simulink model "task2_book"  (R2017a)
settings: Solver=VariableStepAuto  StartTime=0.0  StopTime=400  MaxStep=1e-4*w_base  RelTol=1e-3
settings Model: Creator=Oskar  LastModifiedBy=Callum

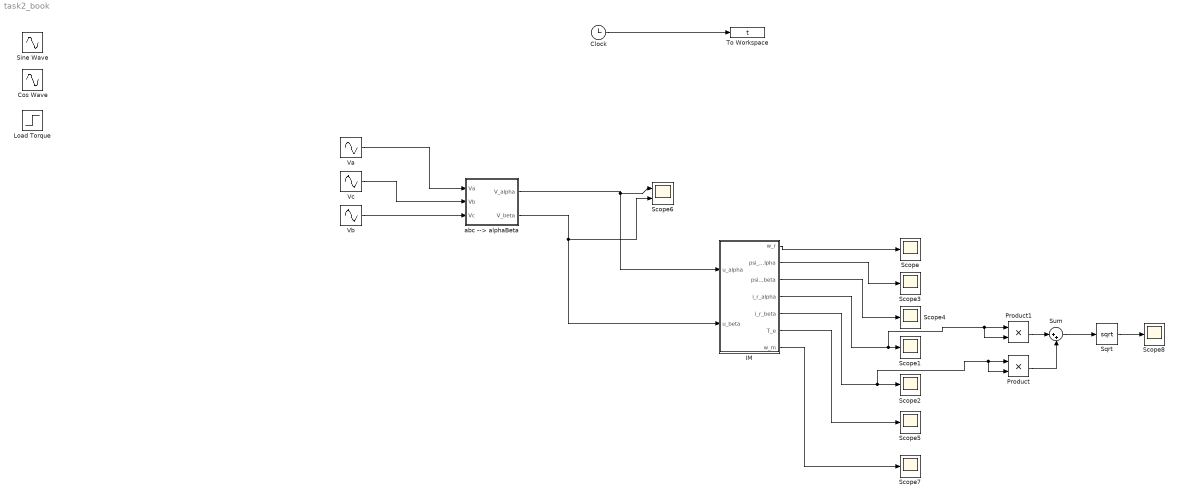
== system task2_book ==
  Clock : Clock
  Cos Wave : Sin  Phase=pi/2  SampleTime=0
  IM : Subsystem  mask{RR=0.02, RS=0.04, LM=2, Ls=0.2, J=100, p=1, b_w1=0.8, b_w2=0}
      mask prompts: RR "Rr [p.u]"; RS "Rs [p.u]"; LM "Lm [p.u]"; Ls "Ls [p.u]"; J "J [p.u]"
  Load Torque : Step  Time=0.3  After=0.3  SampleTime=0
  Product : Product
  Product1 : Product
  Scope{,1..5,7..8} (8 alike) : Scope
  Scope6 : Scope  NumInputPorts=2
  Sine Wave : Sin  SampleTime=0
  Sqrt : Sqrt  SaturateOnIntegerOverflow=on
  Sum : Sum  Inputs=|++
  To Workspace : ToWorkspace  VariableName=t
      settings: MaxDataPoints=10000000
  Va : Sin  Amplitude=sqrt(2)  SampleTime=0
  Vb : Sin  Amplitude=sqrt(2)  Phase=2*pi/3  SampleTime=0
  Vc : Sin  Amplitude=sqrt(2)  Phase=4*pi/3  SampleTime=0
  abc --> alphaBeta : Subsystem
  wires:
  IM/1(w_r) -> Scope/1
  IM/4(i_r_alpha) -> Product1/2, Product1/1, Scope1/1
  IM/5(i_r_beta) -> Product/2, Product/1, Scope2/1
  IM/2(psi_r_alpha) -> Scope3/1
  IM/3(psi_r_beta) -> Scope4/1
  IM/6(T_e) -> Scope5/1
  Va/1 -> abc --> alphaBeta/1(Va)
  abc --> alphaBeta/1(V_alpha) -> Scope6/1, IM/1(u_alpha)
  abc --> alphaBeta/2(V_beta) -> Scope6/2, IM/2(u_beta)
  Vc/1 -> abc --> alphaBeta/2(Vb)
  Vb/1 -> abc --> alphaBeta/3(Vc)
  Clock/1 -> To Workspace/1
  IM/7(w_m) -> Scope7/1
  Product/1 -> Sum/2
  Product1/1 -> Sum/1
  Sum/1 -> Sqrt/1
  Sqrt/1 -> Scope8/1

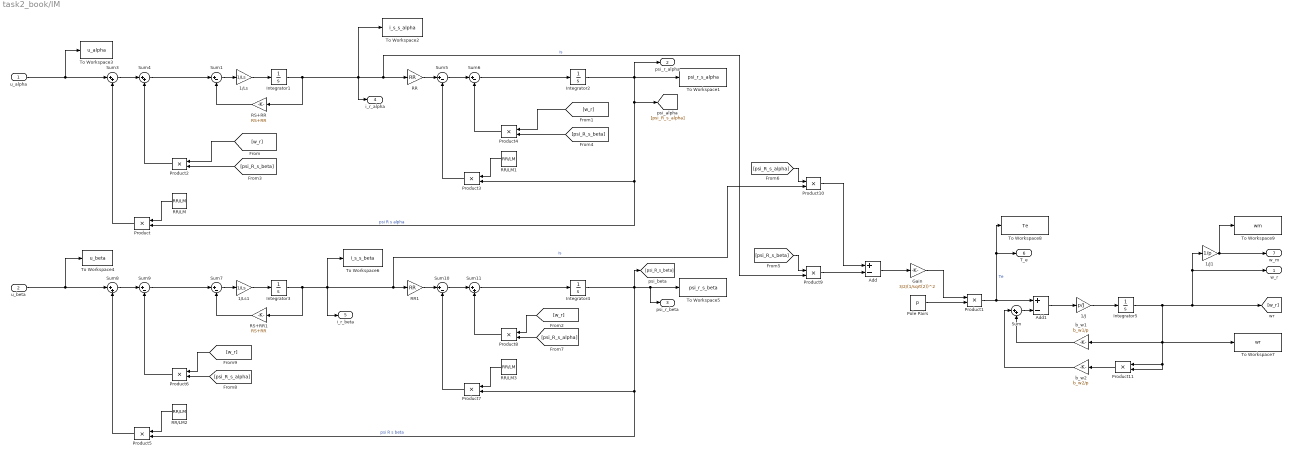
== system task2_book/IM ==
  u_alpha : Inport
  u_beta : Inport  Port=2
  1/J : Gain  Gain=p/J
  1/J1 : Gain  Gain=1/p
  1/Ls : Gain  Gain=1/Ls
  1/Ls1 : Gain  Gain=1/Ls
  Add : Sum  Inputs=+-
  Add1 : Sum  Inputs=+-
  Gain : Gain  Gain=3/2/(1/sqrt(2))^2
  Integrator{1..5} (5 alike) : Integrator
  Pole Pairs : Constant  Value=p
  Product{,1..11} (12 alike) : Product  SaturateOnIntegerOverflow=on  InputSameDT=on  OutDataTypeStr=Inherit: Same as first input
  RR : Gain  Gain=RR
  RR/LM{,1..3} (4 alike) : Constant  Value=RR/LM
  RR1 : Gain  Gain=RR
  RS+RR : Gain  Gain=RS+RR
  RS+RR1 : Gain  Gain=RS+RR
  Sum{,3..4,8,11} (5 alike) : Sum  Inputs=|++
  Sum{1,5..7,9..10} (6 alike) : Sum  Inputs=|+-
  To Workspace1 : ToWorkspace  VariableName=psi_r_s_alpha
      settings: MaxDataPoints=100000
  To Workspace2 : ToWorkspace  VariableName=i_s_s_alpha
      settings: MaxDataPoints=100000
  To Workspace3 : ToWorkspace  VariableName=u_alpha
      settings: MaxDataPoints=100000
  To Workspace4 : ToWorkspace  VariableName=u_beta
      settings: MaxDataPoints=100000
  To Workspace5 : ToWorkspace  VariableName=psi_r_s_beta
      settings: MaxDataPoints=100000
  To Workspace6 : ToWorkspace  VariableName=i_s_s_beta
      settings: MaxDataPoints=100000
  To Workspace7 : ToWorkspace  VariableName=wr
      settings: MaxDataPoints=100000
  To Workspace8 : ToWorkspace  VariableName=Te
      settings: MaxDataPoints=100000
  To Workspace9 : ToWorkspace  VariableName=wm
      settings: MaxDataPoints=100000
  b_w1 : Gain  Gain=b_w1/p
  b_w2 : Gain  Gain=b_w2/p
  w_r : Outport
  psi_r_alpha : Outport  Port=2
  psi_r_beta : Outport  Port=3
  i_r_alpha : Outport  Port=4
  i_r_beta : Outport  Port=5
  T_e : Outport  Port=6
  w_m : Outport  Port=7
  wires:
  RR/LM1/1 -> Product3/1
  Product3/1 -> Sum5/2
  [psi_R_s_alpha] -> Product8/2
  1/Ls/1 -> Integrator1/1
  1/J/1 -> Integrator5/1
  Pole Pairs/1 -> Product1/2
  Add1/1 -> 1/J/1
  Sum1/1 -> 1/Ls/1
  Sum3/1 -> Sum4/1
  Sum4/1 -> Sum1/1
  Integrator2/1 -> psi_r_alpha/1, [psi_R_s_alpha], Product/2, Product3/2, To Workspace1/1  "psi R s alpha"
  RR/LM/1 -> Product/1
  Product10/1 -> Add/1
  Product9/1 -> Add/2
  Sum5/1 -> Sum6/1
  [psi_R_s_beta] -> Product2/2
  [w_r] -> Product2/1
  [w_r] -> Product6/1
  Product/1 -> Sum3/2
  Product1/1 -> To Workspace8/1, T_e/1, Add1/1  "Te"
  [w_r] -> Product8/1
  Sum6/1 -> Integrator2/1
  Add/1 -> Gain/1
  Product5/1 -> Sum8/2
  Sum11/1 -> Integrator4/1
  Integrator3/1 -> i_r_beta/1, Product10/2, RR1/1, To Workspace6/1, RS+RR1/1  "is"
  RR/LM3/1 -> Product7/1
  Sum9/1 -> Sum7/1
  RS+RR1/1 -> Sum7/2
  1/Ls1/1 -> Integrator3/1
  Sum8/1 -> Sum9/1
  Integrator4/1 -> [psi_R_s_beta], Product5/2, Product7/2, psi_r_beta/1, To Workspace5/1  "psi R s beta"
  RR1/1 -> Sum10/1
  Product8/1 -> Sum11/2
  u_beta/1 -> To Workspace4/1, Sum8/1
  Product6/1 -> Sum9/2
  Product7/1 -> Sum10/2
  Sum10/1 -> Sum11/1
  RR/LM2/1 -> Product5/1
  Sum7/1 -> 1/Ls1/1
  [psi_R_s_beta] -> Product9/1
  Integrator1/1 -> i_r_alpha/1, Product9/2, RR/1, To Workspace2/1, RS+RR/1  "is"
  Product4/1 -> Sum6/2
  u_alpha/1 -> Sum3/1, To Workspace3/1
  Gain/1 -> Product1/1
  [w_r] -> Product4/1
  [psi_R_s_alpha] -> Product10/1
  [psi_R_s_alpha] -> Product6/2
  [psi_R_s_beta] -> Product4/2
  RR/1 -> Sum5/1
  RS+RR/1 -> Sum1/2
  Product2/1 -> Sum4/2
  Sum/1 -> Add1/2
  b_w1/1 -> Sum/2
  b_w2/1 -> Sum/1
  Product11/1 -> b_w2/1
  Integrator5/1 -> 1/J1/1, w_r/1, [w_r], Product11/2, Product11/1, b_w1/1, To Workspace7/1
  1/J1/1 -> To Workspace9/1, w_m/1

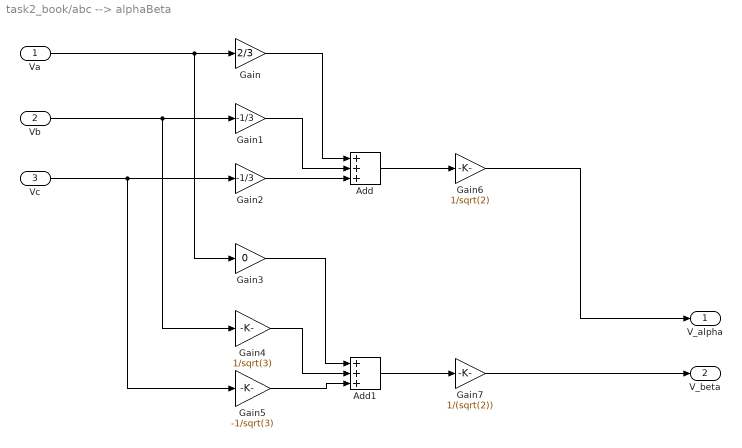
== system task2_book/abc --> alphaBeta ==
  Va : Inport
  Vb : Inport  Port=2
  Vc : Inport  Port=3
  Add : Sum  Inputs=+++
  Add1 : Sum  Inputs=+++
  Gain : Gain  Gain=2/3
  Gain1 : Gain  Gain=-1/3
  Gain2 : Gain  Gain=-1/3
  Gain3 : Gain  Gain=0
  Gain4 : Gain  Gain=1/sqrt(3)
  Gain5 : Gain  Gain=-1/sqrt(3)
  Gain6 : Gain  Gain=1/sqrt(2)
  Gain7 : Gain  Gain=1/(sqrt(2))
  V_alpha : Outport
  V_beta : Outport  Port=2
  wires:
  Add/1 -> Gain6/1
  Va/1 -> Gain3/1, Gain/1
  Vc/1 -> Gain5/1, Gain2/1
  Vb/1 -> Gain4/1, Gain1/1
  Gain3/1 -> Add1/1
  Gain6/1 -> V_alpha/1
  Gain7/1 -> V_beta/1
  Add1/1 -> Gain7/1
  Gain1/1 -> Add/2
  Gain/1 -> Add/1
  Gain5/1 -> Add1/3
  Gain2/1 -> Add/3
  Gain4/1 -> Add1/2
